simulink model "task_3_2"  (R2023a)
settings: Solver=VariableStepAuto  StartTime=0.0  StopTime=100  RelTol=1e-8
settings Model: Creator=user  LastModifiedBy=user

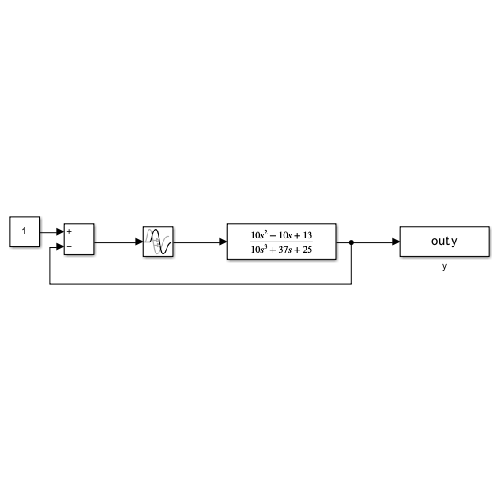
[thumbnail: Simulink's stored preview of the top-level diagram]
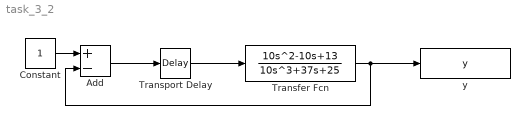
== system task_3_2 ==
  Add : Sum  Inputs=+-
  Constant : Constant  SampleTime=-1
  Transfer Fcn : TransferFcn  Numerator=[10, -10, 13]  Denominator=[10, 0, 37, 25]
  Transport Delay : TransportDelay  DelayTime=0.8  BufferSize=3072
  y : ToWorkspace  VariableName=y  SaveFormat=Timeseries  SampleTime=-1
  wires:
  Transport Delay/1 -> Transfer Fcn/1
  Transfer Fcn/1 -> Add/2, y/1
  Constant/1 -> Add/1
  Add/1 -> Transport Delay/1
